simulink model "lliController"  (R2020b)
settings: Solver=FixedStepAuto  StartTime=0.0  StopTime=5.0  FixedStep=.0002  RelTol=1e-3
libraries: simulink x1
settings Model: Creator=Frienddo  LastModifiedBy=Frienddo

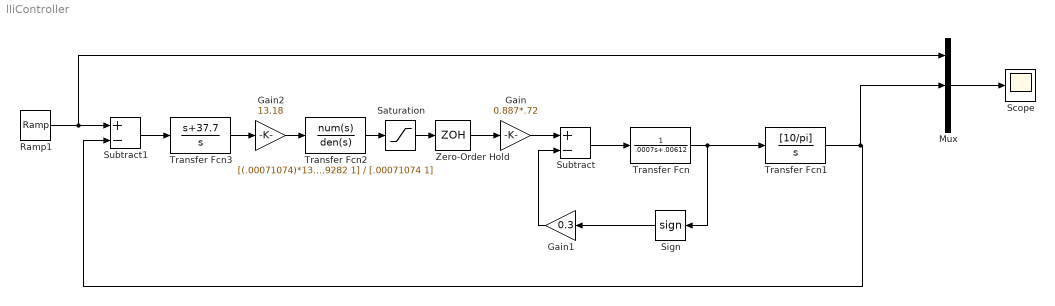
== system lliController ==
  Gain : Gain  Gain=0.887*.72
  Gain1 : Gain  Gain=0.3
  Gain2 : Gain  Gain=13.18
  Mux : Mux  Inputs=3
  Ramp1 : simulink/Sources/Ramp  slope=1  start=0  InitialOutput=0
  Saturation : Saturate  UpperLimit=3  LowerLimit=-3
  Scope : Scope
  Sign : Signum
  Subtract : Sum  Inputs=+-
  Subtract1 : Sum  Inputs=+-
  Transfer Fcn : TransferFcn  Denominator=[.0007 .00612]
  Transfer Fcn1 : TransferFcn  Numerator=[10/pi]  Denominator=[1 0]
  Transfer Fcn2 : TransferFcn  Numerator=[(.00071074)*13.9282 1]  Denominator=[.00071074 1]
  Transfer Fcn3 : TransferFcn  Numerator=[1 37.7]  Denominator=[1 0]
  Zero-Order Hold : ZeroOrderHold  SampleTime=.0002
  wires:
  Saturation/1 -> Zero-Order Hold/1
  Gain/1 -> Subtract/1
  Subtract/1 -> Transfer Fcn/1
  Transfer Fcn/1 -> Sign/1, Transfer Fcn1/1
  Sign/1 -> Gain1/1
  Gain1/1 -> Subtract/2
  Transfer Fcn2/1 -> Saturation/1
  Zero-Order Hold/1 -> Gain/1
  Transfer Fcn1/1 -> Mux/2, Subtract1/2
  Mux/1 -> Scope/1
  Ramp1/1 -> Mux/1, Subtract1/1
  Gain2/1 -> Transfer Fcn2/1
  Subtract1/1 -> Transfer Fcn3/1
  Transfer Fcn3/1 -> Gain2/1
